simulink model "ab"  (R2023b)
settings: configuration reference "VTOLConfiguration" (kept outside this file)
undefined symbols (not defined in the file): airspeed, CityMission, control, controlParams, ControlSampleTime, CriticalTiltAngle, ddx, ddy, ddz, DiscIntNeverNeededParam, dx, dy, dz, Earth, env, F, FixedWingMission, flightState, fractalcoef, FSState, FWControlParams, HoverMission, iniRoll, initPitch, iniYaw, Light, MIL, p, pitch, q, r, R_LOOKAHEAD, ReferenceFilterDen, ReferenceFilterNum, roll, SensorAAFiltDen, SensorAAFiltNum, tiltIni, TiltScheduleRate, TransitionMission, uavParam, UAVSampleTime, vIni, Vt, WGS84, windVel, X, xGround, Y, yaw, yGround, Z, zGround
libraries: slpidlib x37, simulink x10, uavalgslib x6, mbdriLib x4, robotcorelib x3, aerolibasang x2, aerolibwind2 x2, sharedtransform x2, simulink_extras x2, shared6dof x1, aerolibatmos2 x1, sensorgpslib x1
(part 2 of 7)

== system ab/Autopilot/Multicopter Controller/Subsystem ==
  inTransition : Inport
  States : Inport  Port=2
  Reference : Inport  Port=3
  Bus Selector : BusSelector  OutputSignals=ypr
  Bus Selector1 : BusSelector  OutputSignals=ypr,Euler
  NOT : Logic  Operator=NOT  IconShape=distinctive  AllPortsSameDT=off  OutDataTypeStr=boolean
  Scope{,1..3} (4 alike) : Scope
  Selector : Selector  InputPortWidth=3  IndexOptions=Index vector (dialog)  Indices=[1]  OutputSizes=1
  Switch : Switch  Criteria=u2 > Threshold  SaturateOnIntegerOverflow=off  InputSameDT=off
  Triggered Subsystem : Subsystem  TreatAsAtomicUnit=on
  Yaw Reference : Outport
  wires:
  inTransition/1 -> Triggered Subsystem/Trigger, NOT/1
  States/1 -> Bus Selector1/1, Bus Selector/1
  Bus Selector/1 -> Selector/1  "<ypr>"
  Selector/1 -> Triggered Subsystem/1(YawHold)
  NOT/1 -> Switch/2
  Triggered Subsystem/1(Reference) -> Switch/3, Scope1/1  "Stable"
  Switch/1 -> Scope/1, Yaw Reference/1
  Bus Selector1/1 -> Scope2/1  "<ypr>"
  Bus Selector1/2 -> Scope3/1  "<Euler>"
  Reference/1 -> Switch/1

== system ab/Autopilot/Tilt Scheduler/Back Transition Scheduler ==
  Tilt Schedule : Inport
  FlightMode : Inport  Port=2
  States : Inport  Port=3
  Add : Sum  Inputs=+-
  Bus Selector : BusSelector  OutputSignals=Vb
  Constant1 : Constant  Value=flightState.BackTransition
  Constant6 : Constant  Value=0
  Equal1 : RelationalOperator  Operator===  OutDataTypeStr=boolean  RndMeth=Simplest  InputSameDT=off
  Saturation : Saturate  UpperLimit=pi/4  LowerLimit=-pi/4
  Selector : Selector  InputPortWidth=3  IndexOptions=Index vector (dialog)  Indices=[1]  OutputSizes=1
  Switch2 : Switch  Threshold=1  SaturateOnIntegerOverflow=off  InputSameDT=off
  Vx Controller : slpidlib/PID Controller  Controller=P  Form=Parallel  TimeDomain=Discrete-time  UseExternalTs=off  SampleTime=0.005  IntegratorMethod=Forward Euler  FilterMethod=Forward Euler  ControllerParametersSource=internal  P=controlParams.P_BACK  I=0  UseKiTs=off  D=0.0379422021775223  N=1.96946409823213  UseFilter=on  TunerSelectOption=Transfer Function Based (PID Tuner App)  InitialConditionSource=internal  InitialConditionForIntegrator=0  InitialConditionForFilter=0  DifferentiatorICPrevScaledInput=0  ExternalReset=none  TrackingMode=off  Kt=1  LimitOutput=off  SatLimitsSource=internal  UpperSaturationLimit=inf  LowerSaturationLimit=-inf  LinearizeAsGain=on  AntiWindupMode=none  Kb=1  LimitIntegrator=off  UpperIntegratorSaturationLimit=inf  LowerIntegratorSaturationLimit=-inf  POutMin=[]  POutMax=[]  IOutMin=[]  IOutMax=[]  DOutMin=[]  DOutMax=[]  NOutMin=[]  NOutMax=[]  SumOutMin=[]  SumOutMax=[]  SaturationOutMin=[]  SaturationOutMax=[]  PParamMin=[]  PParamMax=[]  IParamMin=[]  IParamMax=[]  DParamMin=[]  DParamMax=[]  NParamMin=[]  NParamMax=[]  KbParamMin=[]  KbParamMax=[]  KtParamMin=[]  KtParamMax=[]  KbOutMin=[]  KbOutMax=[]  KtOutMin=[]  KtOutMax=[]  IntegratorOutMin=[]  IntegratorOutMax=[]  FilterOutMin=[]  FilterOutMax=[]  SumI1OutMin=[]  SumI1OutMax=[]  SumI2OutMin=[]  SumI2OutMax=[]  SumI3OutMin=[]  SumI3OutMax=[]  SumI4OutMin=[]  SumI4OutMax=[]  SumDOutMin=[]  SumDOutMax=[]  DifferentiatorOutMin=[]  DifferentiatorOutMax=[]  FilterDiffOutCoefMin=[]  FilterDiffOutCoefMax=[]  ReciprocalOutMin=[]  ReciprocalOutMax=[]  SumDenOutMin=[]  SumDenOutMax=[]  SumNumOutMin=[]  SumNumOutMax=[]  DivideOutMin=[]  DivideOutMax=[]  UdiffTsProdOutMin=[]  UdiffTsProdOutMax=[]  NTsProdOutMin=[]  NTsProdOutMax=[]  UintegralTsProdOutMin=[]  UintegralTsProdOutMax=[]  UngainTsProdOutMin=[]  UngainTsProdOutMax=[]  ClampingZeroOutDataTypeStr=Inherit: Inherit via back propagation  ClampingZeroOutMin=[]  ClampingZeroOutMax=[]  FilterDenConstantOutDataTypeStr=Inherit: Inherit via back propagation  FilterDenConstantOutMin=[]  FilterDenConstantOutMax=[]  PCopyOutDataTypeStr=Inherit: Inherit via back propagation  PCopyOutMin=[]  PCopyOutMax=[]  NCopyOutDataTypeStr=Inherit: Inherit via back propagation  NCopyOutMin=[]  NCopyOutMax=[]  IntegratorContinuousStateAttributes=''  IntegratorStateMustResolveToSignalObject=off  IntegratorRTWStateStorageClass=Auto  FilterContinuousStateAttributes=''  FilterStateMustResolveToSignalObject=off  FilterRTWStateStorageClass=Auto  ParallelPVariant=InternalParameters  IdealPVariant=Disabled  IVariant=Disabled  DVariant=Disabled  IntegratorVariant=Disabled  SatVariant=Disabled  AWVariant=Disabled  PCopyVariant=Disabled  TRVariant=Disabled  FdbkBlocksVariant=Forward  IdealPFdbkVariant=Disabled  SatFdbkVariant=Disabled  DerivativeFilterVariant=Disabled  NVariant=Disabled  NCopyVariant=Disabled_SignalSpec  FilterICVariant=Disabled  IntegratorICVariant=Disabled  ExternalResetVariant=Disabled  TRSumVariant=Passthrough  SumFdbkVariant=Disabled  SumVariant=Passthrough_P  TsampFilterVariant=InternalTs  TsampNgainVariant=Passthrough  TsampIntegralVariant=Disabled_SignalSpec  ExternalSaturationOutDataTypeStr=Inherit: Same as second input
  TiltAngle : Outport
  wires:
  States/1 -> Bus Selector/1
  Add/1 -> Vx Controller/1
  Equal1/1 -> Switch2/2
  Bus Selector/1 -> Selector/1  "<Vb>"
  FlightMode/1 -> Equal1/1
  Constant1/1 -> Equal1/2
  Constant6/1 -> Add/1
  Selector/1 -> Add/2
  Vx Controller/1 -> Saturation/1
  Saturation/1 -> Switch2/1
  Tilt Schedule/1 -> Switch2/3
  Switch2/1 -> TiltAngle/1

== system ab/Autopilot/Tilt Scheduler/Forward Transition Scheduler ==
  FlightMode : Inport
  Constant : Constant  Value=pi/2
  Constant2 : Constant  Value=0
  Constant3 : Constant  Value=CriticalTiltAngle
  Constant4 : Constant  Value=flightState.Transition
  Constant5 : Constant  Value=TiltScheduleRate
  Equal : RelationalOperator  Operator===  OutDataTypeStr=boolean  RndMeth=Simplest  InputSameDT=off
  Integrator : Integrator  ExternalReset=either  LimitOutput=on  UpperSaturationLimit=Inf  LowerSaturationLimit=0
  LessThanOrEqual : RelationalOperator  Operator=<=  OutDataTypeStr=boolean  RndMeth=Simplest  InputSameDT=off
  Switch : Switch  Criteria=u2 > Threshold  SaturateOnIntegerOverflow=off  InputSameDT=off
  Switch1 : Switch  Criteria=u2 > Threshold  SaturateOnIntegerOverflow=off  InputSameDT=off
  FlightState : Outport
  Tilt Schedule : Outport  Port=2
  tag scope: ModeFlag=global
  wires:
  FlightMode/1 -> FlightState/1, Equal/2
  [ModeFlag] -> Switch1/2, Integrator/2
  Integrator/1 -> Switch/1, LessThanOrEqual/1
  LessThanOrEqual/1 -> Switch/2
  Equal/1 -> [ModeFlag]
  Constant3/1 -> LessThanOrEqual/2
  Switch1/1 -> Integrator/1
  Constant5/1 -> Switch1/1
  Constant2/1 -> Switch1/3
  Constant4/1 -> Equal/1
  Constant/1 -> Switch/3
  Switch/1 -> Tilt Schedule/1

== system ab/Digital Twin/Force and Moments/Aerodynamic Drag ==
  DCM_be : Inport
  Vb : Inport  Port=2
  Constant : Constant  Value=windVel
  Constant1 : Constant  Value=uavParam.aero.dragCoeffMov
  calcDragVector : MATLAB Function  TreatAsAtomicUnit=on
  gain : Gain  Gain=-1
  relative air velocity (body frame) : Sum
  wind (body frame) : Product  Multiplication=Matrix(*)
  F_d : Outport
  wires:
  Vb/1 -> gain/1
  calcDragVector/1(dragVec) -> F_d/1
  relative air velocity (body frame)/1 -> calcDragVector/1(airVel)
  gain/1 -> relative air velocity (body frame)/2
  Constant1/1 -> calcDragVector/2(dragCoeff)
  DCM_be/1 -> wind (body frame)/1
  Constant/1 -> wind (body frame)/2
  wind (body frame)/1 -> relative air velocity (body frame)/1

== system ab/Digital Twin/Force and Moments/Aerodynamic Forces ==
  Wind_e : Inport
  Rho : Inport  Port=2
  CtrlSurfaces : Inport  Port=3
  UAVState : Inport  Port=4
  Bus Selector2 : BusSelector  OutputSignals=Ve,Euler,pqr
  Compute Air Data : Subsystem  TreatAsAtomicUnit=on  VariantControl=use_aerospace_blocks == 1
  Compute Body Frame Forces and Moments : Subsystem
  Rotate Vw : Subsystem
  Vair : Sum  Inputs=-+  InputSameDT=on  SaturateOnIntegerOverflow=on  OutDataTypeStr=Inherit: Same as first input
  AirData : Outport  VectorParamsAs1DForOutWhenUnconnected=off
  F : Outport  Port=2
  M : Outport  Port=3
  wires:
  Bus Selector2/1 -> Vair/2  "<Ve>"
  UAVState/1 -> Bus Selector2/1
  Compute Body Frame Forces and Moments/1(F_b) -> F/1
  Wind_e/1 -> Vair/1
  CtrlSurfaces/1 -> Compute Body Frame Forces and Moments/2(CtrlSurfaces)
  Compute Air Data/1(AirData) -> AirData/1, Compute Body Frame Forces and Moments/1(AirData)
  Bus Selector2/3 -> Compute Body Frame Forces and Moments/3(p,q,r)  "<pqr>"
  Compute Body Frame Forces and Moments/2(M_b) -> M/1
  Rotate Vw/1(Vb) -> Compute Air Data/1(Vb)
  Rho/1 -> Compute Air Data/2(Rho)
  Bus Selector2/2 -> Rotate Vw/2(Euler)  "<Euler>"
  Vair/1 -> Rotate Vw/1(Vw)

== system ab/Digital Twin/Force and Moments/Gravity ==
  DCM_be : Inport
  Constant : Constant  Value=[0 0 uavParam.aero.g]'
  Gain : Gain  Gain=uavParam.geom.mass
  Matrix Multiply : Product  Multiplication=Matrix(*)
  F_g : Outport
  wires:
  Matrix Multiply/1 -> Gain/1
  Constant/1 -> Matrix Multiply/2
  DCM_be/1 -> Matrix Multiply/1
  Gain/1 -> F_g/1

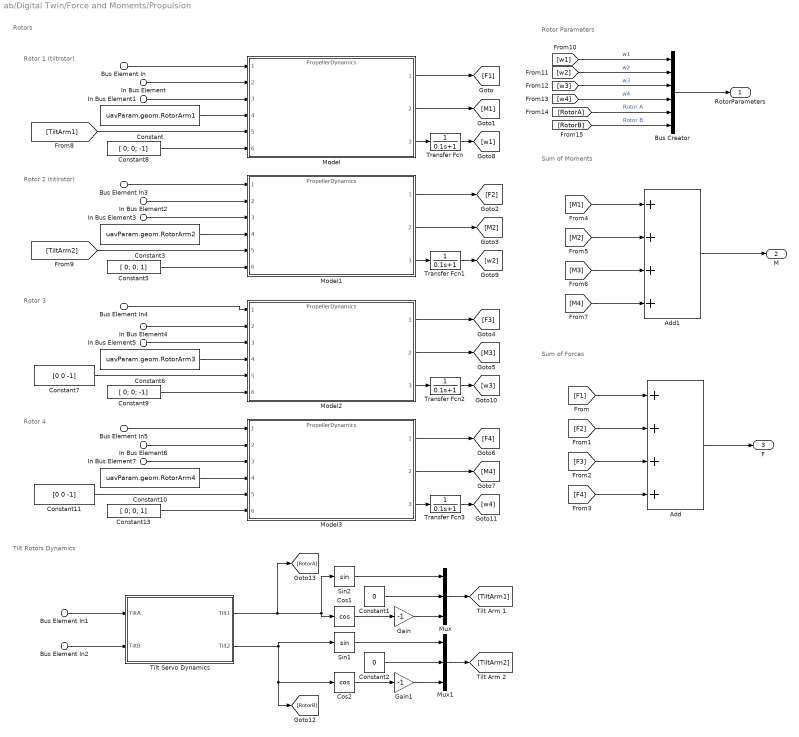
== system ab/Digital Twin/Force and Moments/Propulsion ==
  note: Tilt Rotors Dynamics
  note: Sum of Moments
  note: Rotor 1
      | (tiltrotor)
  note: Rotors
  note: Rotor 2
      | (titlrotor)
  note: Rotor 3
  note: Rotor 4
  note: Sum of Forces
  note: Rotor Parameters
  Bus Element In : Inport  PortName=Actuator  Element=w1
  Bus Element In1 : Inport  PortName=Actuator  Element=Tilt1
  Bus Element In2 : Inport  PortName=Actuator  Element=Tilt2
  Bus Element In3 : Inport  PortName=Actuator  Element=w2
  Bus Element In5 : Inport  PortName=Actuator  Element=w4
  Bus Element In4 : Inport  PortName=Actuator  Element=w3
  In Bus Element{,2,4,6} (4 alike) : Inport  Port=2  PortName=States  Element=Vb
  In Bus Element{1,3,5,7} (4 alike) : Inport  Port=2  PortName=States  Element=pqr
  Add : Sum  Inputs=++++
  Add1 : Sum  Inputs=++++
  Bus Creator : BusCreator  Inputs=6
  Constant : Constant  Value=uavParam.geom.RotorArm1
  Constant1 : Constant  Value=0
  Constant10 : Constant  Value=uavParam.geom.RotorArm4
  Constant11 : Constant  Value=[0 0 -1]
  Constant13 : Constant  Value=[ 0; 0; 1]
  Constant2 : Constant  Value=0
  Constant3 : Constant  Value=uavParam.geom.RotorArm2
  Constant5 : Constant  Value=[ 0; 0; 1]
  Constant6 : Constant  Value=uavParam.geom.RotorArm3
  Constant7 : Constant  Value=[0 0 -1]
  Constant8 : Constant  Value=[ 0; 0; -1]
  Constant9 : Constant  Value=[ 0; 0; -1]
  Cos1 : Trigonometry  Operator=cos
  Cos2 : Trigonometry  Operator=cos
  Gain : Gain  Gain=-1
  Gain1 : Gain  Gain=-1
  Model{,1..3} (4 alike) : ModelReference  ModelNameDialog=PropellerDynamics.slx  ModelReferenceVersion=3.9
  Mux : Mux  Inputs=3
  Mux1 : Mux  Inputs=3
  Sin1 : Trigonometry
  Sin2 : Trigonometry
  Tilt Servo Dynamics : Subsystem
  Transfer Fcn{,1..3} (4 alike) : TransferFcn  Denominator=[0.1 1]
  RotorParameters : Outport
  M : Outport  Port=2
  F : Outport  Port=3
  wires:
  In Bus Element/1 -> Model/2
  In Bus Element1/1 -> Model/3
  Constant/1 -> Model/4
  Sin2/1 -> Mux/1
  Cos1/1 -> Gain/1
  Constant1/1 -> Mux/2
  Gain/1 -> Mux/3
  Mux/1 -> [TiltArm1]
  Cos2/1 -> Gain1/1
  Sin1/1 -> Mux1/1
  Constant2/1 -> Mux1/2
  Mux1/1 -> [TiltArm2]
  [TiltArm1] -> Model/5
  Add/1 -> F/1
  Gain1/1 -> Mux1/3
  Constant8/1 -> Model/6
  Model/1 -> [F1]
  Model/2 -> [M1]
  Model1/1 -> [F2]
  In Bus Element2/1 -> Model1/2
  Constant3/1 -> Model1/4
  Constant5/1 -> Model1/6
  [TiltArm2] -> Model1/5
  In Bus Element3/1 -> Model1/3
  Model1/2 -> [M2]
  Model2/1 -> [F3]
  In Bus Element4/1 -> Model2/2
  Constant6/1 -> Model2/4
  Constant9/1 -> Model2/6
  Constant7/1 -> Model2/5
  In Bus Element5/1 -> Model2/3
  Model2/2 -> [M3]
  Model3/1 -> [F4]
  In Bus Element6/1 -> Model3/2
  Constant10/1 -> Model3/4
  Constant13/1 -> Model3/6
  Constant11/1 -> Model3/5
  In Bus Element7/1 -> Model3/3
  Model3/2 -> [M4]
  [F1] -> Add/1
  [F2] -> Add/2
  [F3] -> Add/3
  [F4] -> Add/4
  [M4] -> Add1/4
  Add1/1 -> M/1
  [M3] -> Add1/3
  [M2] -> Add1/2
  [M1] -> Add1/1
  Model/3 -> Transfer Fcn/1
  Model1/3 -> Transfer Fcn1/1
  Model2/3 -> Transfer Fcn2/1
  Model3/3 -> Transfer Fcn3/1
  [w1] -> Bus Creator/1  "w1"
  [w2] -> Bus Creator/2  "w2"
  [w3] -> Bus Creator/3  "w3"
  [w4] -> Bus Creator/4  "w4"
  Bus Creator/1 -> RotorParameters/1
  [RotorA] -> Bus Creator/5  "Rotor A"
  [RotorB] -> Bus Creator/6  "Rotor B"
  Bus Element In/1 -> Model/1
  Bus Element In3/1 -> Model1/1
  Bus Element In4/1 -> Model2/1
  Bus Element In5/1 -> Model3/1
  Tilt Servo Dynamics/1(Tilt1) -> Cos1/1, Sin2/1, [RotorA]
  Tilt Servo Dynamics/2(Tilt2) -> Sin1/1, Cos2/1, [RotorB]
  Bus Element In1/1 -> Tilt Servo Dynamics/1(TiltA)
  Bus Element In2/1 -> Tilt Servo Dynamics/2(TiltB)
  Transfer Fcn/1 -> [w1]
  Transfer Fcn1/1 -> [w2]
  Transfer Fcn2/1 -> [w3]
  Transfer Fcn3/1 -> [w4]

== system ab/Digital Twin/Force and Moments/Weather Model ==
  AirData : Inport
  Xe : Inport  Port=2
  Euler : Inport  Port=3
  Simple Model : Subsystem  VariantControl=Wind==0
  Weather Model : Subsystem  VariantControl=Wind==1
  Wind_e : Outport
  Rho : Outport  Port=2

== system ab/Digital Twin/Variant Subsystem/No Sensors ==
  Bus Element In9 : Inport  PortName=UAVStates  Element=Ve
  Bus Element In11 : Inport  PortName=UAVStates  Element=Ve
  Bus Element In2 : Inport  PortName=UAVStates  Element=Xe
  Bus Element In3 : Inport  PortName=UAVStates  Element=Euler
  Bus Element In8 : Inport  PortName=UAVStates  Element=Euler
  Bus Element In4 : Inport  PortName=UAVStates  Element=DCMbe
  Bus Element In5 : Inport  PortName=UAVStates  Element=pqr
  Bus Element In6 : Inport  PortName=UAVStates  Element=Vb
  Bus Element In7 : Inport  PortName=UAVStates  Element=Abb
  Bus Element In10 : Inport  PortName=UAVStates  Element=RotorParameters
  Bus Element In : Inport  PortName=UAVStates  Element=airspeed
  Bus Element In12 : Inport  PortName=UAVStates  Element=gndspeed
  Bus Element In1 : Inport  PortName=UAVStates  Element=course
  Bus Creator : BusCreator  Inputs=14
  Direction Cosine Matrix to Quaternions1 : sharedtransform/Direction Cosine Matrix  to Quaternions  aMode=0  action=None  tolerance=eps(2)
      settings: LibrarySourceBlock=|
      | aerolibtransform2/Direction Cosine Matrix
      | to Quaternions
  MATLAB Function : MATLAB Function  TreatAsAtomicUnit=on
  SensorData : Outport
  wires:
  Bus Element In8/1 -> MATLAB Function/1(euler)  "Euler"
  Bus Creator/1 -> SensorData/1
  Bus Element In5/1 -> Bus Creator/8  "pqr"
  Bus Element In2/1 -> Bus Creator/4  "Xe"
  MATLAB Function/1(ypr) -> Bus Creator/13
  Bus Element In9/1 -> Bus Creator/5  "Ve"
  Bus Element In/1 -> Bus Creator/3  "airspeed"
  Bus Element In4/1 -> Bus Creator/6, Direction Cosine Matrix to Quaternions1/1  "DCMbe"
  Direction Cosine Matrix to Quaternions1/1 -> Bus Creator/7
  Bus Element In6/1 -> Bus Creator/9  "Vb"
  Bus Element In7/1 -> Bus Creator/10  "Abb"
  Bus Element In10/1 -> Bus Creator/12  "RotorParameters"
  Bus Element In3/1 -> Bus Creator/11  "Euler"
  Bus Element In11/1 -> Bus Creator/14  "Ve_ground"
  Bus Element In12/1 -> Bus Creator/2  "gndspeed"
  Bus Element In1/1 -> Bus Creator/1  "course"

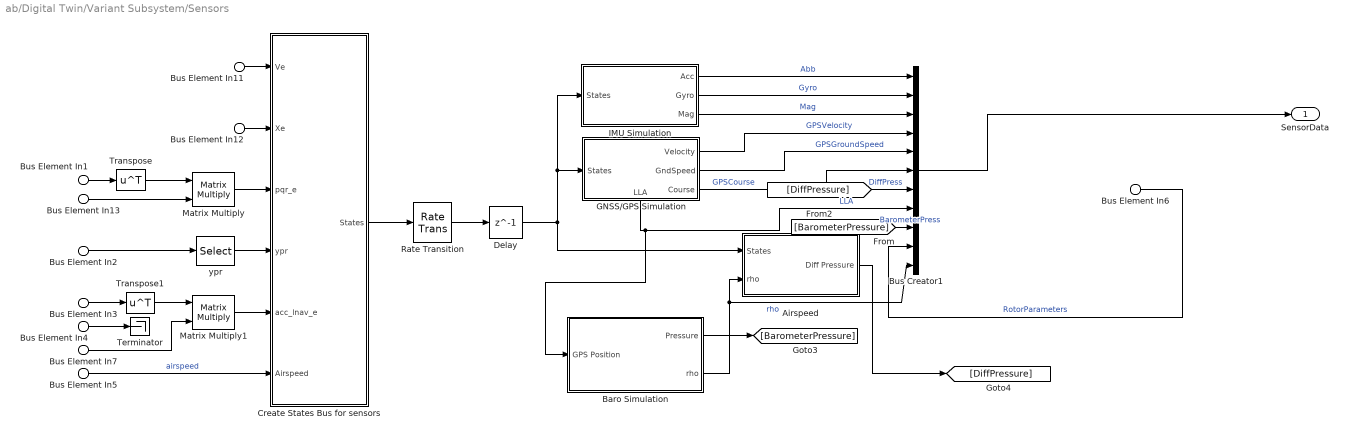
== system ab/Digital Twin/Variant Subsystem/Sensors ==
  Bus Element In11 : Inport  PortName=UAVStates  Element=Ve
  Bus Element In12 : Inport  PortName=UAVStates  Element=Xe
  Bus Element In13 : Inport  PortName=UAVStates  Element=pqr
  Bus Element In1 : Inport  PortName=UAVStates  Element=DCMbe
  Bus Element In3 : Inport  PortName=UAVStates  Element=DCMbe
  Bus Element In2 : Inport  PortName=UAVStates  Element=Euler
  Bus Element In4 : Inport  PortName=UAVStates  Element=Abb
  Bus Element In5 : Inport  PortName=UAVStates  Element=airspeed
  Bus Element In6 : Inport  PortName=UAVStates  Element=RotorParameters
  Bus Element In7 : Inport  PortName=UAVStates  Element=Abe
  " Baro Simulation" : Subsystem
  Airspeed : Subsystem
  Bus Creator1 : BusCreator  Inputs=11
  Create States Bus for sensors : Subsystem
  Delay : Delay  DelayLength=1
  GNSS/GPS Simulation : Subsystem
      settings: PortSchema="{\"entries\":[{\"content\":{\"sides\":[{\"content\":{\"connectorIds\":[\"In1\"]},\"type\":\"ConnectorPlacement.EquallySpacedRectSide\",\"uuid\":\"4934e8ff-5d4b-4e11-968d-c23bd62383a0\"},{\"content\":{\"connectorIds\":[\"Out1\",\"Out2\",\"Out3\"],\"side\":\"RIGHT\"},\"type\":\"ConnectorPlacement.EquallySpacedRectSide\",\"uuid\":\"9ec8bc0a-2d3c-4dca-835c-010ac29b6ebc\"},{\"content\":{\"connectorIds\":[],\"side\":\"TOP\"},\"type\":\"ConnectorPlacement.EquallySpacedRectSide\",\"uuid\":\"04f09eb4-1bd9-450e-b951-47054bdd92ad\"},{\"content\":{\"connectorIds\":[\"Out4\"],\"side\":\"BOTTOM\"},\"type\":\"ConnectorPlacement.EquallySpacedRectSide\",\"uuid\":\"54bba437-6d13-4ada-8e8d-b8e04495ee78\"}]},\"type\":\"ConnectorPlacement.EquallySpacedConnector\",\"uuid\":\"9a5920cf-a58d-4c98-839b-fbac94edbe7e\"}],\"packageUris\":[\"http://schema.mathworks.com/mf0/Connector/R2020b\"],\"version\":\"1.0\"}"
  IMU Simulation : Subsystem
  Matrix Multiply : Product  Multiplication=Matrix(*)
  Matrix Multiply1 : Product  Multiplication=Matrix(*)
  Rate Transition : RateTransition  OutPortSampleTime=0.001
  Terminator : Terminator
  Transpose : Math  Operator=transpose
  Transpose1 : Math  Operator=transpose
  ypr : Selector  InputPortWidth=3  IndexOptions=Index vector (dialog)  Indices=[3 2 1]  OutputSizes=1
  SensorData : Outport
  wires:
  GNSS/GPS Simulation/2(GndSpeed) -> Bus Creator1/5  "GPSGroundSpeed"
  Rate Transition/1 -> Delay/1
  Bus Element In1/1 -> Transpose/1
  Bus Element In13/1 -> Matrix Multiply/2
  IMU Simulation/1(Acc) -> Bus Creator1/1  "Abb"
  IMU Simulation/2(Gyro) -> Bus Creator1/2  "Gyro"
  [BarometerPressure] -> Bus Creator1/9  "BarometerPress"
  Bus Element In11/1 -> Create States Bus for sensors/1(Ve)
  GNSS/GPS Simulation/3(Course) -> Bus Creator1/6  "GPSCourse"
  " Baro Simulation"/2(rho) -> Bus Creator1/11, Airspeed/2(rho)  "rho"
  GNSS/GPS Simulation/4(LLA) -> Bus Creator1/8, " Baro Simulation"/1(GPS Position)  "LLA"
  Transpose1/1 -> Matrix Multiply1/1
  Delay/1 -> IMU Simulation/1(States), GNSS/GPS Simulation/1(States), Airspeed/1(States)
  Bus Element In6/1 -> Bus Creator1/10  "RotorParameters"
  [DiffPressure] -> Bus Creator1/7  "DiffPress"
  Bus Element In12/1 -> Create States Bus for sensors/2(Xe)
  Create States Bus for sensors/1(States) -> Rate Transition/1
  " Baro Simulation"/1(Pressure) -> [BarometerPressure]
  Bus Element In5/1 -> Create States Bus for sensors/6(Airspeed)  "airspeed"
  Matrix Multiply/1 -> Create States Bus for sensors/3(pqr_e)
  GNSS/GPS Simulation/1(Velocity) -> Bus Creator1/4  "GPSVelocity"
  Bus Element In2/1 -> ypr/1
  IMU Simulation/3(Mag) -> Bus Creator1/3  "Mag"
  Bus Element In7/1 -> Matrix Multiply1/2
  Airspeed/1(Diff Pressure) -> [DiffPressure]
  Matrix Multiply1/1 -> Create States Bus for sensors/5(acc_lnav_e)
  ypr/1 -> Create States Bus for sensors/4(ypr)
  Bus Element In3/1 -> Transpose1/1
  Transpose/1 -> Matrix Multiply/1
  Bus Element In4/1 -> Terminator/1
  Bus Creator1/1 -> SensorData/1

== system ab/Estimator/Estimation Filter/Airspeed Filter ==
  DiffPress : Inport
  rho : Inport  Port=2
  Constant : Constant  Value=0.5
  Divide : Product  Inputs=*/
  Product : Product
  Sqrt : Sqrt
  airspeed : Outport
  wires:
  Constant/1 -> Product/2
  rho/1 -> Product/1
  Product/1 -> Divide/2
  DiffPress/1 -> Divide/1
  Divide/1 -> Sqrt/1
  Sqrt/1 -> airspeed/1

== system ab/Estimator/Estimation Filter/LLA2Local ==
  LLA : Inport
  Constant1 : Constant  Value=0
  Demux1 : Demux  Outputs=2
  LLA to Flat Earth1 : aerolibtransform2/LLA to Flat Earth  units=Metric (MKS)  ptype=Earth (WGS84)  F=1/298.257223563  R=6378137  refPosPort=off  LL0=[0 0]  psi=0
  Xe : Outport
  wires:
  Constant1/1 -> LLA to Flat Earth1/3
  Demux1/1 -> LLA to Flat Earth1/1
  Demux1/2 -> LLA to Flat Earth1/2
  LLA to Flat Earth1/1 -> Xe/1  "Xe"
  LLA/1 -> Demux1/1

== system ab/Ground Control Station/Get Flight Mission/noQGC ==
  note: uavPathManagerBus type
  No Mission : Constant  Value=struct('mode',0,'position',[0 0 0]','params',[0;0;0;0]);  OutDataTypeStr=Bus: doubleUavPathManager
  Variant Source : VariantSource
  Waypoints : Constant  Value=FixedWingMission  OutDataTypeStr=Bus: doubleUavPathManager  SampleTime=-1
  Waypoints1 : Constant  Value=HoverMission  OutDataTypeStr=Bus: doubleUavPathManager  SampleTime=-1
  Waypoints2 : Constant  Value=TransitionMission  OutDataTypeStr=Bus: doubleUavPathManager  SampleTime=-1
  Waypoints3 : Constant  Value=CityMission  OutDataTypeStr=Bus: doubleUavPathManager  SampleTime=-1
  Mission : Outport
  wires:
  Waypoints/1 -> Variant Source/2
  Waypoints1/1 -> Variant Source/3
  Variant Source/1 -> Mission/1
  Waypoints2/1 -> Variant Source/4
  No Mission/1 -> Variant Source/1
  Waypoints3/1 -> Variant Source/5

== system ab/Guidance Test Bench/ControlType/Guidance Testbench ==
  Global Mission : Inport
  Aircraft States : Inport  Port=2
  Control Rate Transition : Subsystem
  Guidance Logic : Subsystem  VariantControl=guidanceType==1
  HoverCmds : Outport
  FixedWingSP : Outport  Port=2
  AACSP : Outport  Port=3
  ctrlMode : Outport  Port=4
  FlightMode : Outport  Port=5
  wires:
  Aircraft States/1 -> Guidance Logic/1(UAVState)
  Global Mission/1 -> Guidance Logic/2(GCSCommands)
  Guidance Logic/1(HoverGuidance) -> Control Rate Transition/1("1 ")
  Guidance Logic/2(FixedWingSP) -> Control Rate Transition/2(In2)
  Guidance Logic/3(AACSP) -> Control Rate Transition/3(In3)
  Guidance Logic/4(ctrlMode) -> Control Rate Transition/4(In4)
  Guidance Logic/5(FlightMode) -> Control Rate Transition/5(In5)
  Control Rate Transition/1(Out1) -> HoverCmds/1
  Control Rate Transition/2(Out2) -> FixedWingSP/1
  Control Rate Transition/3(Out3) -> AACSP/1
  Control Rate Transition/4(Out4) -> ctrlMode/1
  Control Rate Transition/5(Out5) -> FlightMode/1

== system ab/Guidance Test Bench/ControlType/Manual Control ==
  note: Commanded Altitude (m)
  note: Commanded Y (m)
  note: Fixed Wing Aerodynamics
  note: Commanded X (m)
  note: Fixed Wing
  note: Hover
  note: Flight Mode
  note: Transition
  note: Commanded Course
  note: Commanded Altitude
  note: Commanded Airspeed (m)
  note: Back Transition
  note: Fixed Wing Commands
  note: Hover Commands
  Global Mission : Inport
  Aircraft States : Inport  Port=2
  Command Interface : Subsystem
  Slider1 : SliderBlock  LabelPosition=Hide  ScaleMax=50  TickInterval=5
  Slider2 : SliderBlock  LabelPosition=Hide  ScaleMin=-30  ScaleMax=30  TickInterval=5
  Slider3 : SliderBlock  LabelPosition=Hide  ScaleMin=-30  ScaleMax=30  TickInterval=5
  Slider4 : SliderBlock  LabelPosition=Hide  ScaleMax=3  TickInterval=1
  Slider5 : SliderBlock  LabelPosition=Hide  ScaleMin=-30  ScaleMax=30  TickInterval=5
  Slider6 : SliderBlock  LabelPosition=Hide  ScaleMin=-100  TickInterval=10
  Slider7 : SliderBlock  LabelPosition=Hide  ScaleMin=10  ScaleMax=30  TickInterval=5
  Toggle Switch1 : ToggleSwitchBlock  LabelPosition=Hide
      settings: Values={{'Off', 'On'}, [0 1]}
  HoverCmds : Outport
  FixedWingSP : Outport  Port=2
  AACSP : Outport  Port=3
  ctrlMode : Outport  Port=4
  FlightMode : Outport  Port=5
  wires:
  Global Mission/1 -> Command Interface/1(Global Mission)
  Aircraft States/1 -> Command Interface/2(Aircraft States)
  Command Interface/1(ctrlMode) -> ctrlMode/1
  Command Interface/2(FixedWingSP) -> FixedWingSP/1
  Command Interface/3(AACSP) -> AACSP/1
  Command Interface/4(PositionCmds) -> HoverCmds/1
  Command Interface/5(FlightMode) -> FlightMode/1

== system ab/Guidance Test Bench/Reference Tracking /Fixed Wing Reference ==
  AAC Commands : Inport
  States : Inport  Port=2
  Bus Creator1 : BusCreator  Inputs=2
  Bus Creator2 : BusCreator  Inputs=3
  Bus Selector : BusSelector  OutputSignals=airspeed,Xe,course
  Bus Selector3 : BusSelector  OutputSignals=airspeed,altitude,course
  Gain : Gain  Gain=-1
  Mux1 : Mux  Inputs=3
  Selector : Selector  InputPortWidth=3  IndexOptions=Index vector (dialog)  Indices=3  OutputSizes=1
  To Workspace1 : ToWorkspace  VariableName=FixedWingCmdFdbk  SaveFormat=Structure With Time  SampleTime=-1
  wires:
  Selector/1 -> Gain/1
  Bus Selector3/1 -> Mux1/1  "<airspeed>"
  Bus Selector/1 -> Bus Creator2/1  "<airspeed>"
  Bus Selector3/2 -> Mux1/2  "<altitude>"
  Bus Selector/3 -> Bus Creator2/3  "<course>"
  Mux1/1 -> Bus Creator1/1
  Bus Creator1/1 -> To Workspace1/1
  Bus Selector3/3 -> Mux1/3  "<course>"
  Gain/1 -> Bus Creator2/2  "altitude"
  Bus Creator2/1 -> Bus Creator1/2
  AAC Commands/1 -> Bus Selector3/1
  Bus Selector/2 -> Selector/1  "<Xe>"
  States/1 -> Bus Selector/1

== system ab/Guidance Test Bench/Reference Tracking /Hover Reference ==
  Position Command : Inport
  Position Reference : Inport  Port=2
  Bus Creator : BusCreator  Inputs=2
  Bus Selector1 : BusSelector  OutputSignals=Xe  OutputAsBus=on
  Bus Selector2 : BusSelector  OutputSignals=X,Y,Z
  Mux : Mux  Inputs=3
  To Workspace : ToWorkspace  VariableName=PositionCmdFdbk  SaveFormat=Structure With Time  SampleTime=-1
  wires:
  Position Reference/1 -> Bus Selector1/1
  Bus Selector2/3 -> Mux/3  "<Z>"
  Bus Selector2/1 -> Mux/1  "<X>"
  Bus Selector1/1 -> Bus Creator/2
  Bus Creator/1 -> To Workspace/1
  Bus Selector2/2 -> Mux/2  "<Y>"
  Mux/1 -> Bus Creator/1
  Position Command/1 -> Bus Selector2/1

== system ab/Guidance Test Bench/Reference Tracking /Transition Reference ==
  States : Inport
  Bus Creator : BusCreator  Inputs=4
  Bus Selector4 : BusSelector  OutputSignals=airspeed,RotorParameters.Rotor A,Euler,Xe
  Gain : Gain  Gain=-1
  Selector : Selector  InputPortWidth=3  IndexOptions=Index vector (dialog)  Indices=[2]  OutputSizes=1
  Selector1 : Selector  InputPortWidth=3  IndexOptions=Index vector (dialog)  Indices=[3]  OutputSizes=1
  To Workspace1 : ToWorkspace  VariableName=TransitionFeedback  SaveFormat=Structure With Time  SampleTime=-1
  wires:
  States/1 -> Bus Selector4/1
  Bus Selector4/3 -> Selector/1  "<Euler>"
  Bus Selector4/4 -> Selector1/1  "<Xe>"
  Selector1/1 -> Gain/1
  Bus Selector4/1 -> Bus Creator/1  "<airspeed>"
  Selector/1 -> Bus Creator/3  "pitch"
  Gain/1 -> Bus Creator/4  "altitude"
  Bus Selector4/2 -> Bus Creator/2  "<Rotor A>"
  Bus Creator/1 -> To Workspace1/1

== system ab/Visualization/Photorealistic/Prepare UAV Data ==
  UAVState : Inport
  Bus Selector1 : BusSelector  OutputSignals=x,y,z,yaw,pitch,roll
  Gain{,1..3} (4 alike) : Gain  Gain=-1
  Mux : Mux  Inputs=3
  Mux1 : Mux  Inputs=3
  Translation : Outport
  Rotation : Outport  Port=2
  wires:
  UAVState/1 -> Bus Selector1/1
  Mux/1 -> Translation/1
  Mux1/1 -> Rotation/1  "EulerZYX"
  Bus Selector1/4 -> Gain3/1  "<yaw>"
  Bus Selector1/5 -> Gain2/1  "<pitch>"
  Bus Selector1/6 -> Mux1/3  "<roll>"
  Bus Selector1/3 -> Gain/1  "<z>"
  Bus Selector1/2 -> Gain1/1  "<y>"
  Bus Selector1/1 -> Mux/1  "<x>"
  Gain/1 -> Mux/3
  Gain1/1 -> Mux/2
  Gain2/1 -> Mux1/2
  Gain3/1 -> Mux1/1

== system ab/Visualization/Visualization/Subsystem ==
  <Xe> : Inport
  <q> : Inport  Port=2
  RotorA : Inport  Port=3
  RotorB : Inport  Port=4
  Constant : Constant  Value=0
  Constant1 : Constant  Value=0
  Gain : Gain  Gain=0
  Gain1 : Gain  Gain=-1
  Gain2 : Gain  Gain=-1
  MATLAB System : MATLABSystem  System=exampleHelperTiltRotorAnimator  SampleTime=0.05
      mask Type: exampleHelperTiltRotorAnimator
      mask Display:
      | disp('exampleHelperTiltRotorAnimator');
      | port_label('input',1,'position');
      | port_label('input',2,'orientation');
      | port_label('input',3,'rotorAngles');
  Mux : Mux
  Reshape : Reshape  OutputDimensionality=Customize  OutputDimensions=[1,4]
  Reshape1 : Reshape  OutputDimensionality=Customize  OutputDimensions=[1,4]
  Reshape2 : Reshape  OutputDimensionality=Customize  OutputDimensions=[1,3]
  wires:
  Gain1/1 -> Mux/1
  Constant1/1 -> Mux/4
  Gain2/1 -> Mux/2
  Reshape1/1 -> MATLAB System/3
  Mux/1 -> Reshape1/1
  RotorA/1 -> Gain1/1
  <Xe>/1 -> Gain/1
  Constant/1 -> Mux/3
  RotorB/1 -> Gain2/1
  <q>/1 -> Reshape/1
  Reshape2/1 -> MATLAB System/1
  Reshape/1 -> MATLAB System/2
  Gain/1 -> Reshape2/1

== system ab/Autopilot/Fixed Wing Controller/Fixed Wing Controller Simulation/AER from Path Manager ==
  In1 : Inport
  Enable : EnablePort
  Out1 : Outport
  wires:
  In1/1 -> Out1/1

== system ab/Autopilot/Fixed Wing Controller/Fixed Wing Controller Simulation/Airspeed-Altitude Controller ==
  note: Airspeed and altitude are controlled independently
      | by ignoring their coupled dynamics.
  Airspeed SP : Inport
  Altitude SP : Inport  Port=2
  Climb Rate SP : Inport  Port=3
  Airspeed : Inport  Port=4
  xyz : Inport  Port=5
  vxyz : Inport  Port=6
  Enable : EnablePort  ShowOutputPort=on
  Airspeed Controller : slpidlib/PID Controller  Controller=PID  Form=Parallel  TimeDomain=Discrete-time  UseExternalTs=off  SampleTime=ControlSampleTime  IntegratorMethod=Trapezoidal  FilterMethod=Forward Euler  ControllerParametersSource=internal  P=FWControlParams.P_AIRSPD  I=FWControlParams.I_AIRSPD  UseKiTs=off  D=FWControlParams.D_AIRSPD  N=FWControlParams.N_AIRSPD  UseFilter=on  TunerSelectOption=Transfer Function Based (PID Tuner App)  InitialConditionSource=internal  InitialConditionForIntegrator=0  InitialConditionForFilter=0  DifferentiatorICPrevScaledInput=0  ExternalReset=none  TrackingMode=off  Kt=1  LimitOutput=off  SatLimitsSource=internal  UpperSaturationLimit=Inf  LowerSaturationLimit=0  LinearizeAsGain=on  AntiWindupMode=clamping  Kb=1  LimitIntegrator=off  UpperIntegratorSaturationLimit=inf  LowerIntegratorSaturationLimit=-inf  POutMin=[]  POutMax=[]  IOutMin=[]  IOutMax=[]  DOutMin=[]  DOutMax=[]  NOutMin=[]  NOutMax=[]  SumOutMin=[]  SumOutMax=[]  SaturationOutMin=[]  SaturationOutMax=[]  PParamMin=[]  PParamMax=[]  IParamMin=[]  IParamMax=[]  DParamMin=[]  DParamMax=[]  NParamMin=[]  NParamMax=[]  KbParamMin=[]  KbParamMax=[]  KtParamMin=[]  KtParamMax=[]  KbOutMin=[]  KbOutMax=[]  KtOutMin=[]  KtOutMax=[]  IntegratorOutMin=[]  IntegratorOutMax=[]  FilterOutMin=[]  FilterOutMax=[]  SumI1OutMin=[]  SumI1OutMax=[]  SumI2OutMin=[]  SumI2OutMax=[]  SumI3OutMin=[]  SumI3OutMax=[]  SumI4OutMin=[]  SumI4OutMax=[]  SumDOutMin=[]  SumDOutMax=[]  DifferentiatorOutMin=[]  DifferentiatorOutMax=[]  FilterDiffOutCoefMin=[]  FilterDiffOutCoefMax=[]  ReciprocalOutMin=[]  ReciprocalOutMax=[]  SumDenOutMin=[]  SumDenOutMax=[]  SumNumOutMin=[]  SumNumOutMax=[]  DivideOutMin=[]  DivideOutMax=[]  UdiffTsProdOutMin=[]  UdiffTsProdOutMax=[]  NTsProdOutMin=[]  NTsProdOutMax=[]  UintegralTsProdOutMin=[]  UintegralTsProdOutMax=[]  UngainTsProdOutMin=[]  UngainTsProdOutMax=[]  ClampingZeroOutDataTypeStr=Inherit: Inherit via back propagation  ClampingZeroOutMin=[]  ClampingZeroOutMax=[]  FilterDenConstantOutDataTypeStr=Inherit: Inherit via back propagation  FilterDenConstantOutMin=[]  FilterDenConstantOutMax=[]  PCopyOutDataTypeStr=Inherit: Inherit via back propagation  PCopyOutMin=[]  PCopyOutMax=[]  NCopyOutDataTypeStr=Inherit: Inherit via back propagation  NCopyOutMin=[]  NCopyOutMax=[]  IntegratorContinuousStateAttributes=''  IntegratorStateMustResolveToSignalObject=off  IntegratorRTWStateStorageClass=Auto  FilterContinuousStateAttributes=''  FilterStateMustResolveToSignalObject=off  FilterRTWStateStorageClass=Auto  ParallelPVariant=InternalParameters  IdealPVariant=Disabled  IVariant=InternalParameters  DVariant=InternalParameters  IntegratorVariant=Discrete  SatVariant=Disabled  AWVariant=Passthrough  PCopyVariant=Disabled  TRVariant=Disabled  FdbkBlocksVariant=Forward  IdealPFdbkVariant=Disabled  SatFdbkVariant=Disabled  DerivativeFilterVariant=ForwardEulerFilter  NVariant=InternalParameters  NCopyVariant=Disabled  FilterICVariant=InternalICsFilter  IntegratorICVariant=InternalICs  ExternalResetVariant=Disabled  TRSumVariant=Passthrough  SumFdbkVariant=Disabled  SumVariant=Sum_PID  TsampFilterVariant=InternalTs  TsampNgainVariant=Passthrough  TsampIntegralVariant=Disabled_SignalSpec  ExternalSaturationOutDataTypeStr=Inherit: Same as second input
  Altitude controller : Subsystem
  Climb Rate SP Merge : Merge
  Climb Rate SP from Guidance : Subsystem  TreatAsAtomicUnit=on
  Compare To Constant : simulink/Logic and Bit Operations/Compare To Constant  relop===  const=uint8(1)  OutDataTypeStr=boolean
  Compare To Constant1 : simulink/Logic and Bit Operations/Compare To Constant  relop===  const=uint8(2)  OutDataTypeStr=boolean
  Mux : Mux  Inputs=2
  Pitch SP Controller : Subsystem
  Scope : Scope
  Scope1 : Scope
  Sum1 : Sum  Inputs=|+-
  Pitch SP : Outport
  Throttle : Outport  Port=2
  wires:
  Airspeed SP/1 -> Mux/1, Sum1/1
  Sum1/1 -> Airspeed Controller/1
  Airspeed/1 -> Sum1/2, Mux/2
  Airspeed Controller/1 -> Scope1/1, Throttle/1
  Altitude SP/1 -> Altitude controller/1(Alt SP)
  xyz/1 -> Altitude controller/2(xyz)
  vxyz/1 -> Pitch SP Controller/2(vxyz)
  Pitch SP Controller/1(Pitch SP) -> Pitch SP/1
  Enable/1 -> Compare To Constant1/1, Compare To Constant/1
  Compare To Constant/1 -> Altitude controller/Enable
  Compare To Constant1/1 -> Climb Rate SP from Guidance/Enable
  Altitude controller/1(Climb Rate SP) -> Climb Rate SP Merge/1
  Climb Rate SP from Guidance/1(Out1) -> Climb Rate SP Merge/2
  Climb Rate SP Merge/1 -> Pitch SP Controller/1(Climb Rate SP)
  Climb Rate SP/1 -> Climb Rate SP from Guidance/1(Climb Rate SP)
  Mux/1 -> Scope/1

== system ab/Autopilot/Fixed Wing Controller/Fixed Wing Controller Simulation/Attitude Controller ==
  YPR SP : Inport
  ypr : Inport  Port=2
  Ang Rate : Inport  Port=3
  Airspeed : Inport  Port=4
  Enable : EnablePort  ShowOutputPort=on
  AER Merge : Merge
  Compare To Constant : simulink/Logic and Bit Operations/Compare To Constant  relop===  const=uint8(1)  OutDataTypeStr=boolean
  Compare To Constant1 : simulink/Logic and Bit Operations/Compare To Constant  relop===  const=uint8(2)  OutDataTypeStr=boolean
  Demux1 : Demux  Outputs=3
  Pitch Roll Controller : Subsystem
  Rudder Heading Controller : Subsystem
  AER : Outport
  wires:
  ypr/1 -> Rudder Heading Controller/2(YPR), Pitch Roll Controller/3(YPR)
  YPR SP/1 -> Demux1/1
  Enable/1 -> Compare To Constant1/1, Compare To Constant/1
  AER Merge/1 -> AER/1
  Compare To Constant/1 -> Pitch Roll Controller/Enable
  Pitch Roll Controller/1(AER) -> AER Merge/1
  Rudder Heading Controller/1(AER) -> AER Merge/2
  Demux1/1 -> Rudder Heading Controller/1(Yaw SP)
  Demux1/2 -> Pitch Roll Controller/1(Pitch SP)
  Demux1/3 -> Pitch Roll Controller/2(Roll SP)
  Ang Rate/1 -> Rudder Heading Controller/3(Ang Rate), Pitch Roll Controller/4(Ang Rate)
  Compare To Constant1/1 -> Rudder Heading Controller/Enable
  Airspeed/1 -> Pitch Roll Controller/5(Airspeed)

== system ab/Autopilot/Fixed Wing Controller/Fixed Wing Controller Simulation/Lateral Guidance Logic ==
  note: S. Park, J. Deyst, and J. P. How, "A New Nonlinear Guidance Logic for Trajectory Tracking," Proceedings of the AIAA Guidance, Navigation and Control Conference, Aug 2004. AIAA-2004-4900.
  Course SP : Inport
  L1 Distance : Inport  Port=2
  course : Inport  Port=3
  gndspeed : Inport  Port=4
  Enable : EnablePort
  MATLAB Function : MATLAB Function  TreatAsAtomicUnit=on  SystemSampleTime=ControlSampleTime
  Terminator : Terminator
  Roll SP : Outport
  wires:
  Course SP/1 -> MATLAB Function/1(courseSP)
  course/1 -> MATLAB Function/2(course)
  MATLAB Function/2(rollSP) -> Roll SP/1
  MATLAB Function/1(lacc) -> Terminator/1
  gndspeed/1 -> MATLAB Function/3(groundSpeed)
  L1 Distance/1 -> MATLAB Function/4(L1)

== system ab/Autopilot/Fixed Wing Controller/Fixed Wing Controller Simulation/Pitch, Airspeed SP from Controller ==
  Pitch SP In : Inport
  Airspeed SP : Inport  Port=2
  Airspeed : Inport  Port=3
  Enable : EnablePort
  Airspeed Controller : slpidlib/PID Controller  Controller=PID  Form=Parallel  TimeDomain=Discrete-time  UseExternalTs=off  SampleTime=ControlSampleTime  IntegratorMethod=Trapezoidal  FilterMethod=Forward Euler  ControllerParametersSource=internal  P=FWControlParams.P_AIRSPD  I=FWControlParams.I_AIRSPD  UseKiTs=off  D=FWControlParams.D_AIRSPD  N=FWControlParams.N_AIRSPD  UseFilter=on  TunerSelectOption=Transfer Function Based (PID Tuner App)  InitialConditionSource=internal  InitialConditionForIntegrator=0  InitialConditionForFilter=0  DifferentiatorICPrevScaledInput=0  ExternalReset=none  TrackingMode=off  Kt=1  LimitOutput=off  SatLimitsSource=internal  UpperSaturationLimit=Inf  LowerSaturationLimit=0  LinearizeAsGain=on  AntiWindupMode=clamping  Kb=1  LimitIntegrator=off  UpperIntegratorSaturationLimit=inf  LowerIntegratorSaturationLimit=-inf  POutMin=[]  POutMax=[]  IOutMin=[]  IOutMax=[]  DOutMin=[]  DOutMax=[]  NOutMin=[]  NOutMax=[]  SumOutMin=[]  SumOutMax=[]  SaturationOutMin=[]  SaturationOutMax=[]  PParamMin=[]  PParamMax=[]  IParamMin=[]  IParamMax=[]  DParamMin=[]  DParamMax=[]  NParamMin=[]  NParamMax=[]  KbParamMin=[]  KbParamMax=[]  KtParamMin=[]  KtParamMax=[]  KbOutMin=[]  KbOutMax=[]  KtOutMin=[]  KtOutMax=[]  IntegratorOutMin=[]  IntegratorOutMax=[]  FilterOutMin=[]  FilterOutMax=[]  SumI1OutMin=[]  SumI1OutMax=[]  SumI2OutMin=[]  SumI2OutMax=[]  SumI3OutMin=[]  SumI3OutMax=[]  SumI4OutMin=[]  SumI4OutMax=[]  SumDOutMin=[]  SumDOutMax=[]  DifferentiatorOutMin=[]  DifferentiatorOutMax=[]  FilterDiffOutCoefMin=[]  FilterDiffOutCoefMax=[]  ReciprocalOutMin=[]  ReciprocalOutMax=[]  SumDenOutMin=[]  SumDenOutMax=[]  SumNumOutMin=[]  SumNumOutMax=[]  DivideOutMin=[]  DivideOutMax=[]  UdiffTsProdOutMin=[]  UdiffTsProdOutMax=[]  NTsProdOutMin=[]  NTsProdOutMax=[]  UintegralTsProdOutMin=[]  UintegralTsProdOutMax=[]  UngainTsProdOutMin=[]  UngainTsProdOutMax=[]  ClampingZeroOutDataTypeStr=Inherit: Inherit via back propagation  ClampingZeroOutMin=[]  ClampingZeroOutMax=[]  FilterDenConstantOutDataTypeStr=Inherit: Inherit via back propagation  FilterDenConstantOutMin=[]  FilterDenConstantOutMax=[]  PCopyOutDataTypeStr=Inherit: Inherit via back propagation  PCopyOutMin=[]  PCopyOutMax=[]  NCopyOutDataTypeStr=Inherit: Inherit via back propagation  NCopyOutMin=[]  NCopyOutMax=[]  IntegratorContinuousStateAttributes=''  IntegratorStateMustResolveToSignalObject=off  IntegratorRTWStateStorageClass=Auto  FilterContinuousStateAttributes=''  FilterStateMustResolveToSignalObject=off  FilterRTWStateStorageClass=Auto  ParallelPVariant=InternalParameters  IdealPVariant=Disabled  IVariant=InternalParameters  DVariant=InternalParameters  IntegratorVariant=Discrete  SatVariant=Disabled  AWVariant=Passthrough  PCopyVariant=Disabled  TRVariant=Disabled  FdbkBlocksVariant=Forward  IdealPFdbkVariant=Disabled  SatFdbkVariant=Disabled  DerivativeFilterVariant=ForwardEulerFilter  NVariant=InternalParameters  NCopyVariant=Disabled  FilterICVariant=InternalICsFilter  IntegratorICVariant=InternalICs  ExternalResetVariant=Disabled  TRSumVariant=Passthrough  SumFdbkVariant=Disabled  SumVariant=Sum_PID  TsampFilterVariant=InternalTs  TsampNgainVariant=Passthrough  TsampIntegralVariant=Disabled_SignalSpec  ExternalSaturationOutDataTypeStr=Inherit: Same as second input
  IC : InitialCondition  Value=0
  Sum1 : Sum  Inputs=|+-
  Pitch SP : Outport
  Throttle : Outport  Port=2
  wires:
  IC/1 -> Pitch SP/1
  Pitch SP In/1 -> IC/1
  Airspeed SP/1 -> Sum1/1
  Sum1/1 -> Airspeed Controller/1
  Airspeed/1 -> Sum1/2
  Airspeed Controller/1 -> Throttle/1

== system ab/Autopilot/Fixed Wing Controller/Fixed Wing Controller Simulation/Roll SP from Path Manager ==
  In1 : Inport
  Enable : EnablePort
  IC : InitialCondition  Value=0
  Out1 : Outport
  wires:
  In1/1 -> IC/1
  IC/1 -> Out1/1

== system ab/Autopilot/Fixed Wing Controller/Fixed Wing Controller Simulation/Subsystem2 ==
  Euler : Inport
  pqr : Inport  Port=2
  Demux : Demux  Outputs=3
  Display : Display
  MATLAB Function : MATLAB Function  TreatAsAtomicUnit=on
  Matrix Multiply : Product  Multiplication=Matrix(*)
  Terminator : Terminator
  Euler Rate : Outport
  wires:
  Demux/1 -> MATLAB Function/1(phi)
  Demux/2 -> MATLAB Function/2(theta)
  MATLAB Function/1(y) -> Matrix Multiply/1
  pqr/1 -> Matrix Multiply/2
  Euler/1 -> Demux/1
  Demux/3 -> Terminator/1
  Matrix Multiply/1 -> Display/1, Euler Rate/1

== system ab/Autopilot/Fixed Wing Controller/Fixed Wing Controller Tuning/AER from Path Manager ==
  In1 : Inport
  Enable : EnablePort
  Out1 : Outport
  wires:
  In1/1 -> Out1/1

== system ab/Autopilot/Fixed Wing Controller/Fixed Wing Controller Tuning/Airspeed-Altitude Controller ==
  note: Airspeed and altitude are controlled independently
      | by ignoring their coupled dynamics.
  Airspeed SP : Inport
  Altitude SP : Inport  Port=2
  Climb Rate SP : Inport  Port=3
  Airspeed : Inport  Port=4
  xyz : Inport  Port=5
  vxyz : Inport  Port=6
  Enable : EnablePort  ShowOutputPort=on
  Airspeed Controller : slpidlib/PID Controller  Controller=PID  Form=Parallel  TimeDomain=Discrete-time  UseExternalTs=off  SampleTime=ControlSampleTime  IntegratorMethod=Trapezoidal  FilterMethod=Forward Euler  ControllerParametersSource=internal  P=40.1166410885074  I=21.6851560041072  UseKiTs=off  D=2.18528545905044  N=172.44752694034  UseFilter=on  TunerSelectOption=Transfer Function Based (PID Tuner App)  InitialConditionSource=internal  InitialConditionForIntegrator=0  InitialConditionForFilter=0  DifferentiatorICPrevScaledInput=0  ExternalReset=none  TrackingMode=off  Kt=1  LimitOutput=off  SatLimitsSource=internal  UpperSaturationLimit=Inf  LowerSaturationLimit=0  LinearizeAsGain=on  AntiWindupMode=clamping  Kb=1  LimitIntegrator=off  UpperIntegratorSaturationLimit=inf  LowerIntegratorSaturationLimit=-inf  POutMin=[]  POutMax=[]  IOutMin=[]  IOutMax=[]  DOutMin=[]  DOutMax=[]  NOutMin=[]  NOutMax=[]  SumOutMin=[]  SumOutMax=[]  SaturationOutMin=[]  SaturationOutMax=[]  PParamMin=[]  PParamMax=[]  IParamMin=[]  IParamMax=[]  DParamMin=[]  DParamMax=[]  NParamMin=[]  NParamMax=[]  KbParamMin=[]  KbParamMax=[]  KtParamMin=[]  KtParamMax=[]  KbOutMin=[]  KbOutMax=[]  KtOutMin=[]  KtOutMax=[]  IntegratorOutMin=[]  IntegratorOutMax=[]  FilterOutMin=[]  FilterOutMax=[]  SumI1OutMin=[]  SumI1OutMax=[]  SumI2OutMin=[]  SumI2OutMax=[]  SumI3OutMin=[]  SumI3OutMax=[]  SumI4OutMin=[]  SumI4OutMax=[]  SumDOutMin=[]  SumDOutMax=[]  DifferentiatorOutMin=[]  DifferentiatorOutMax=[]  FilterDiffOutCoefMin=[]  FilterDiffOutCoefMax=[]  ReciprocalOutMin=[]  ReciprocalOutMax=[]  SumDenOutMin=[]  SumDenOutMax=[]  SumNumOutMin=[]  SumNumOutMax=[]  DivideOutMin=[]  DivideOutMax=[]  UdiffTsProdOutMin=[]  UdiffTsProdOutMax=[]  NTsProdOutMin=[]  NTsProdOutMax=[]  UintegralTsProdOutMin=[]  UintegralTsProdOutMax=[]  UngainTsProdOutMin=[]  UngainTsProdOutMax=[]  ClampingZeroOutDataTypeStr=Inherit: Inherit via back propagation  ClampingZeroOutMin=[]  ClampingZeroOutMax=[]  FilterDenConstantOutDataTypeStr=Inherit: Inherit via back propagation  FilterDenConstantOutMin=[]  FilterDenConstantOutMax=[]  PCopyOutDataTypeStr=Inherit: Inherit via back propagation  PCopyOutMin=[]  PCopyOutMax=[]  NCopyOutDataTypeStr=Inherit: Inherit via back propagation  NCopyOutMin=[]  NCopyOutMax=[]  IntegratorContinuousStateAttributes=''  IntegratorStateMustResolveToSignalObject=off  IntegratorRTWStateStorageClass=Auto  FilterContinuousStateAttributes=''  FilterStateMustResolveToSignalObject=off  FilterRTWStateStorageClass=Auto  ParallelPVariant=InternalParameters  IdealPVariant=Disabled  IVariant=InternalParameters  DVariant=InternalParameters  IntegratorVariant=Discrete  SatVariant=Disabled  AWVariant=Passthrough  PCopyVariant=Disabled  TRVariant=Disabled  FdbkBlocksVariant=Forward  IdealPFdbkVariant=Disabled  SatFdbkVariant=Disabled  DerivativeFilterVariant=ForwardEulerFilter  NVariant=InternalParameters  NCopyVariant=Disabled  FilterICVariant=InternalICsFilter  IntegratorICVariant=InternalICs  ExternalResetVariant=Disabled  TRSumVariant=Passthrough  SumFdbkVariant=Disabled  SumVariant=Sum_PID  TsampFilterVariant=InternalTs  TsampNgainVariant=Passthrough  TsampIntegralVariant=Disabled_SignalSpec  ExternalSaturationOutDataTypeStr=Inherit: Same as second input
  Altitude Controller : Subsystem
  Climb Rate SP Switch : Switch  Criteria=u2 > Threshold  SaturateOnIntegerOverflow=off  InputSameDT=off
  Climb Rate SP from Guidance : Subsystem  TreatAsAtomicUnit=on
  Compare To Constant : simulink/Logic and Bit Operations/Compare To Constant  relop===  const=uint8(1)  OutDataTypeStr=boolean
  Compare To Constant1 : simulink/Logic and Bit Operations/Compare To Constant  relop===  const=uint8(2)  OutDataTypeStr=boolean
  Pitch SP Controller : Subsystem
  Sum1 : Sum  Inputs=|+-
  Pitch SP : Outport
  Throttle : Outport  Port=2
  wires:
  Airspeed SP/1 -> Sum1/1
  Sum1/1 -> Airspeed Controller/1
  Airspeed/1 -> Sum1/2
  Airspeed Controller/1 -> Throttle/1
  Altitude SP/1 -> Altitude Controller/1(Alt SP)
  xyz/1 -> Altitude Controller/2(xyz)
  vxyz/1 -> Pitch SP Controller/2(vxyz)
  Pitch SP Controller/1(Pitch SP) -> Pitch SP/1
  Enable/1 -> Compare To Constant1/1, Compare To Constant/1
  Compare To Constant/1 -> Climb Rate SP Switch/2, Altitude Controller/Enable
  Compare To Constant1/1 -> Climb Rate SP from Guidance/Enable
  Altitude Controller/1(Climb Rate SP) -> Climb Rate SP Switch/1
  Climb Rate SP from Guidance/1(Out1) -> Climb Rate SP Switch/3
  Climb Rate SP Switch/1 -> Pitch SP Controller/1(Climb Rate SP)
  Climb Rate SP/1 -> Climb Rate SP from Guidance/1(Climb Rate SP)

== system ab/Autopilot/Fixed Wing Controller/Fixed Wing Controller Tuning/Attitude Controller ==
  YPR SP : Inport
  ypr : Inport  Port=2
  Ang Rate : Inport  Port=3
  Airspeed : Inport  Port=4
  Enable : EnablePort  ShowOutputPort=on
  AER Switch : Switch  Criteria=u2 > Threshold  SaturateOnIntegerOverflow=off  InputSameDT=off
  Compare To Constant : simulink/Logic and Bit Operations/Compare To Constant  relop===  const=uint8(1)  OutDataTypeStr=boolean
  Compare To Constant1 : simulink/Logic and Bit Operations/Compare To Constant  relop===  const=uint8(2)  OutDataTypeStr=boolean
  Demux1 : Demux  Outputs=3
  Pitch Roll Controller : Subsystem
  Rudder Heading Controller : Subsystem
  AER : Outport
  wires:
  ypr/1 -> Rudder Heading Controller/2(YPR), Pitch Roll Controller/3(YPR)
  YPR SP/1 -> Demux1/1
  Enable/1 -> Compare To Constant1/1, Compare To Constant/1
  AER Switch/1 -> AER/1
  Compare To Constant/1 -> AER Switch/2, Pitch Roll Controller/Enable
  Pitch Roll Controller/1(AER) -> AER Switch/1
  Rudder Heading Controller/1(AER) -> AER Switch/3
  Demux1/1 -> Rudder Heading Controller/1(Yaw SP)
  Demux1/2 -> Pitch Roll Controller/1(Pitch SP)
  Demux1/3 -> Pitch Roll Controller/2(Roll SP)
  Ang Rate/1 -> Rudder Heading Controller/3(Ang Rate), Pitch Roll Controller/4(Ang Rate)
  Compare To Constant1/1 -> Rudder Heading Controller/Enable
  Airspeed/1 -> Pitch Roll Controller/5(Airspeed)

== system ab/Autopilot/Fixed Wing Controller/Fixed Wing Controller Tuning/Lateral Guidance Logic ==
  note: S. Park, J. Deyst, and J. P. How, "A New Nonlinear Guidance Logic for Trajectory Tracking," Proceedings of the AIAA Guidance, Navigation and Control Conference, Aug 2004. AIAA-2004-4900.
  Course SP : Inport
  L1 Distance : Inport  Port=2
  course : Inport  Port=3
  gndspeed : Inport  Port=4
  Enable : EnablePort
  MATLAB Function : MATLAB Function  TreatAsAtomicUnit=on  SystemSampleTime=ControlSampleTime
  Terminator : Terminator
  Roll SP : Outport
  wires:
  Course SP/1 -> MATLAB Function/1(courseSP)
  course/1 -> MATLAB Function/2(course)
  MATLAB Function/2(rollSP) -> Roll SP/1
  MATLAB Function/1(lacc) -> Terminator/1
  gndspeed/1 -> MATLAB Function/3(groundSpeed)
  L1 Distance/1 -> MATLAB Function/4(L1)
